simulink model "PID_loop_exec"  (Simulink 3.00)
libraries: execlib x8

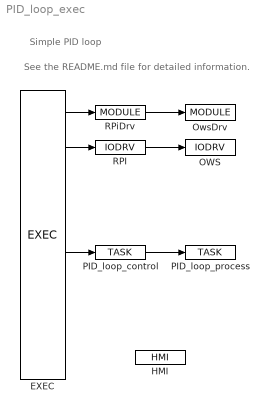
== system PID_loop_exec ==
  note: See the README.md file for detailed information.
  note: Simple PID loop
  EXEC : execlib/EXEC  target=PC - Linux  tick=0.01  ntick0=10  ntick1=50  ntick2=100  ntick3=1200  pri0=5  pri1=9  pri2=13  pri3=18
  HMI : execlib/HMI  IncludeHMI=on  HmiDir=hmi  SourceDir=hmisrc  GenerateWebWatch=on  GenerateRexHMI=on  RedirectToHMI=off  Compression=off
  OWS : execlib/IODRV  module=OwsDrv  classname=OwsDrv  cfgname=pid_loop_owscfg.rio  factor=100  stack=10240  pri=3  timer=off
  OwsDrv : execlib/MODULE
  PID_loop_control : execlib/TASK  factor=1  start=0  stop=1  stack=10240  MDLOPEN=on
  PID_loop_process : execlib/TASK  factor=1  start=1  stop=2  stack=10240  MDLOPEN=on
  RPI : execlib/IODRV  module=RPiDrv  classname=RPiDrv  factor=1  stack=10240  pri=3  timer=off
  RPiDrv : execlib/MODULE
  wires:
  EXEC/1 -> RPiDrv/1
  EXEC/2 -> RPI/1
  EXEC/5 -> PID_loop_control/1
  PID_loop_control/1 -> PID_loop_process/1
  RPI/1 -> OWS/1
  RPiDrv/1 -> OwsDrv/1
